simulink library "SOMANET"  (R2016b)
settings: Solver=VariableStepAuto  StartTime=0.0  StopTime=10.0  RelTol=1e-3
undefined symbols (not defined in the file): currentNominal, SomanetError
libraries: simulink x3, ConfigHandler x1, ElectricPowerMotorCalculator x1, SafetyCheckerSOMANET x1, TuningHandler x1, StatemachineSOMANET x1
settings Model: Creator=Nathan  LastModifiedBy=march

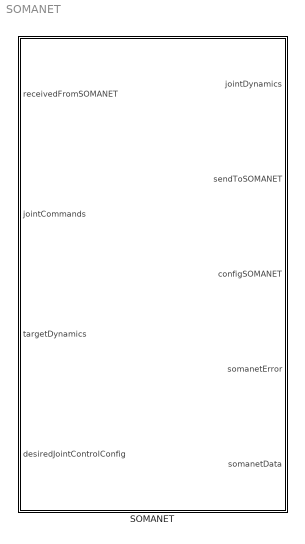
== system SOMANET ==
  SOMANET : Subsystem

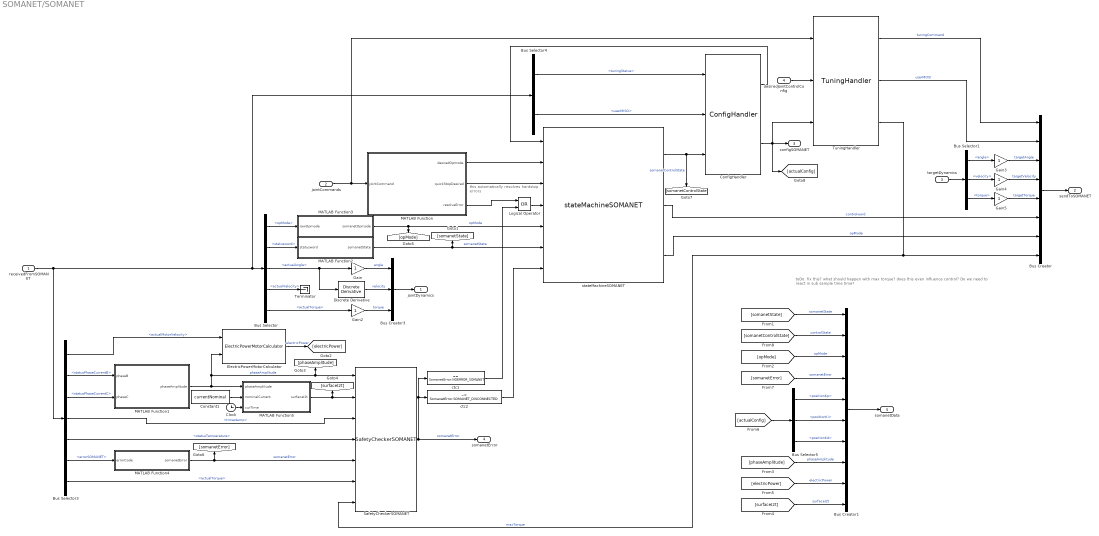
== system SOMANET/SOMANET ==
  note: this automatically resolves hardstop errors
  note: toDo: fix this? what should happen with max torque? does this even influence control? Do we need to react in sub sample time time?
  receivedFromSOMANET : Inport  OutDataTypeStr=Bus: EtherCATReceivedFromSOMANET  BusOutputAsStruct=on
  jointCommands : Inport  Port=2
  targetDynamics : Inport  Port=3  OutDataTypeStr=Bus: JointDynamics  BusOutputAsStruct=on
  desiredJointControlConfig : Inport  Port=4  OutDataTypeStr=Bus: JointControlConfig
  Bus Creator : BusCreator  Inputs=8  OutDataTypeStr=Bus: EtherCATSendToSOMANET  NonVirtualBus=on
  Bus Creator1 : BusCreator  Inputs=10  OutDataTypeStr=Bus: SOMANETData  NonVirtualBus=on
  Bus Creator3 : BusCreator  Inputs=3  OutDataTypeStr=Bus: JointDynamics  NonVirtualBus=on
  Bus Selector : BusSelector  OutputSignals=opMode,statusword,actualAngle,actualVelocity,actualTorque
  Bus Selector1 : BusSelector  OutputSignals=angle,velocity,torque
  Bus Selector3 : BusSelector  OutputSignals=actualMotorVelocity,statusPhaseCurrentB,statusPhaseCurrentC,timestamp,statusTemperature,errorSOMANET,actualTorque
  Bus Selector4 : BusSelector  OutputSignals=tuningStatus,userMISO
  Bus Selector5 : BusSelector  OutputSignals=positionKp,positionKi,positionKd
  Clock : Clock
  ConfigHandler : ConfigHandler/ConfigHandler
  Constant1 : Constant  Value=currentNominal
  Discrete Derivative : simulink/Discrete/Discrete Derivative  gainval=1.0  ICPrevScaledInput=0.0  OutMin=[]  OutMax=[]  OutDataType=fixdt(1, 16)  OutScaling=2^-10  DoSatur=off
  ElectricPowerMotorCalculator : ElectricPowerMotorCalculator/ElectricPowerMotorCalculator
  Gain{,2..5} (5 alike) : Gain
  Logical Operator : Logic  Operator=OR  AllPortsSameDT=off  OutDataTypeStr=boolean
  MATLAB Function : MATLAB Function  TreatAsAtomicUnit=on
  MATLAB Function1 : MATLAB Function  TreatAsAtomicUnit=on
  MATLAB Function2 : MATLAB Function  TreatAsAtomicUnit=on
  MATLAB Function3 : MATLAB Function  TreatAsAtomicUnit=on
  MATLAB Function4 : MATLAB Function  TreatAsAtomicUnit=on
  MATLAB Function5 : MATLAB Function  TreatAsAtomicUnit=on
  SafetyCheckerSOMANET : SafetyCheckerSOMANET/SafetyCheckerSOMANET
  Terminator : Terminator
  TuningHandler : TuningHandler/TuningHandler
  ctc1 : simulink/Logic and Bit Operations/Compare To Constant  relop===  const=SomanetError.NOERROR_SOMANET  OutDataTypeStr=boolean
  ctc2 : simulink/Logic and Bit Operations/Compare To Constant  relop=~=  const=SomanetError.SOMANET_DISCONNECTED  OutDataTypeStr=boolean
  stateMachineSOMANET : StatemachineSOMANET/stateMachineSOMANET
  jointDynamics : Outport  OutDataTypeStr=Bus: JointDynamics
  sendToSOMANET : Outport  Port=2  OutDataTypeStr=Bus: EtherCATSendToSOMANET  BusOutputAsStruct=on
  configSOMANET : Outport  Port=3  OutDataTypeStr=Bus: JointControlConfig  BusOutputAsStruct=on
  somanetError : Outport  Port=4  OutDataTypeStr=Enum: SomanetError
  somanetData : Outport  Port=5  OutDataTypeStr=Bus: SOMANETData
  wires:
  Bus Selector5/3 -> Bus Creator1/7  "<positionKd>"
  Bus Selector5/2 -> Bus Creator1/6  "<positionKi>"
  Bus Selector5/1 -> Bus Creator1/5  "<positionKp>"
  [actualConfig] -> Bus Selector5/1
  Gain5/1 -> Bus Creator/5  "targetTorque"
  Gain3/1 -> Bus Creator/3  "targetAngle"
  Gain4/1 -> Bus Creator/4  "targetVelocity"
  Bus Selector1/3 -> Gain5/1  "<torque>"
  Bus Selector1/1 -> Gain3/1  "<angle>"
  Bus Selector1/2 -> Gain4/1  "<velocity>"
  Gain2/1 -> Bus Creator3/3  "torque"
  Discrete Derivative/1 -> Bus Creator3/2  "velocity"
  Gain/1 -> Bus Creator3/1  "angle"
  Bus Selector/2 -> MATLAB Function2/1(statusword)  "<statusword>"
  Bus Selector/1 -> MATLAB Function3/1(rawOpmode)  "<opMode>"
  ConfigHandler/1 -> stateMachineSOMANET/1
  SafetyCheckerSOMANET/1 -> ctc1/1, ctc2/1, somanetError/1  "somanetError"
  jointCommands/1 -> MATLAB Function/1(jointCommand), TuningHandler/1
  Bus Creator/1 -> sendToSOMANET/1
  receivedFromSOMANET/1 -> Bus Selector4/1, Bus Selector/1, Bus Selector3/1
  TuningHandler/3 -> SafetyCheckerSOMANET/7, Bus Creator/8  "maxTorque"
  MATLAB Function3/1(somanetOpmode) -> [opMode], stateMachineSOMANET/5  "opMode"
  MATLAB Function2/1(somanetState) -> [somanetState], stateMachineSOMANET/6  "somanetState"
  MATLAB Function/1(desiredOpmode) -> stateMachineSOMANET/2
  ctc2/1 -> stateMachineSOMANET/7
  MATLAB Function/2(quickStopDesired) -> stateMachineSOMANET/3
  Bus Creator3/1 -> jointDynamics/1
  Bus Selector/4 -> Terminator/1  "<actualVelocity>"
  Bus Selector/3 -> Gain/1, Discrete Derivative/1  "<actualAngle>"
  targetDynamics/1 -> Bus Selector1/1
  Bus Selector4/1 -> ConfigHandler/1  "<tuningStatus>"
  Bus Selector4/2 -> ConfigHandler/2  "<userMISO>"
  stateMachineSOMANET/1 -> [somanetControlState], ConfigHandler/3  "somanetControlState"
  ConfigHandler/2 -> [actualConfig], configSOMANET/1, TuningHandler/3
  desiredJointControlConfig/1 -> TuningHandler/2
  TuningHandler/1 -> Bus Creator/1  "tuningCommand"
  TuningHandler/2 -> Bus Creator/2  "userMOSI"
  stateMachineSOMANET/2 -> Bus Creator/6  "controlword"
  stateMachineSOMANET/3 -> Bus Creator/7  "opMode"
  Bus Selector/5 -> Gain2/1  "<actualTorque>"
  Bus Selector3/1 -> ElectricPowerMotorCalculator/1  "<actualMotorVelocity>"
  Bus Selector3/2 -> MATLAB Function1/1(phaseB)  "<statusPhaseCurrentB>"
  Bus Selector3/3 -> MATLAB Function1/2(phaseC)  "<statusPhaseCurrentC>"
  Bus Selector3/6 -> MATLAB Function4/1(errorCode)  "<errorSOMANET>"
  MATLAB Function4/1(somanetError) -> SafetyCheckerSOMANET/5, [somanetError]  "somanetError"
  MATLAB Function1/1(phaseAmplitude) -> ElectricPowerMotorCalculator/2, [phaseAmplitude], SafetyCheckerSOMANET/1, MATLAB Function5/1(phaseAmplitude)  "phaseAmplitude"
  Clock/1 -> MATLAB Function5/3(curTime)
  MATLAB Function5/1(surfaceI2t) -> SafetyCheckerSOMANET/2, [surfaceI2t]
  Bus Selector3/4 -> SafetyCheckerSOMANET/3  "<timestamp>"
  Bus Selector3/5 -> SafetyCheckerSOMANET/4  "<statusTemperature>"
  Constant1/1 -> MATLAB Function5/2(nominalCurrent)
  ElectricPowerMotorCalculator/1 -> [electricPower]  "electricPower"
  [somanetState] -> Bus Creator1/1  "somanetState"
  [opMode] -> Bus Creator1/3  "opMode"
  [somanetError] -> Bus Creator1/4  "somanetError"
  [somanetControlState] -> Bus Creator1/2  "controlState"
  [phaseAmplitude] -> Bus Creator1/8  "phaseAmplitude"
  [electricPower] -> Bus Creator1/9  "electricPower"
  [surfaceI2t] -> Bus Creator1/10  "surfaceI2t"
  Bus Creator1/1 -> somanetData/1
  Bus Selector3/7 -> SafetyCheckerSOMANET/6  "<actualTorque>"
  Logical Operator/1 -> stateMachineSOMANET/4
  MATLAB Function/3(resolveError) -> Logical Operator/1
  ctc1/1 -> Logical Operator/2

== matlab function SOMANET/MATLAB Function5 ==
  data: phaseAmplitude input; surfaceI2t output; nominalCurrent input; curTime input
function surfaceI2t = getI2tSurface( phaseAmplitude, nominalCurrent, curTime )
% wrapper for getI2tSurface
surfaceI2t = getI2tSurface(phaseAmplitude, nominalCurrent, curTime);
end

== matlab function SOMANET/MATLAB Function ==
  data: jointCommand input; desiredOpmode output; quickStopDesired output; resolveError output
function [desiredOpmode, quickStopDesired, resolveError] = getSomanetCommands(jointCommand)
% jointCommand should be some enum
% with possible values something like:
%   * torqueControl
%   * positionControl
%   * velocityControl
%   * deactivateMotors
%   * resetError (?)
%   * don't move
% from these commands, the desired control words/opmodes/quick stops/
% whatever can be derived.
% point of this is that the master can be agnostic about the precise
% control mechanism of the somanet
persistent prevOpmode;
if(isempty(prevOpmode))
    prevOpmode = SomanetOpmode.CSTORQUE;
end

switch jointCommand
    case JointCommand.POSITIONCONTROL
        desiredOpmode = SomanetOpmode.CSPOSITION;
        quickStopDesired = 0;
        resolveError = 0;
    case JointCommand.VELOCITYCONTROL
        desiredOpmode = SomanetOpmode.CSVELOCITY;
        quickStopDesired = 0;
        resolveError = 0;
    case JointCommand.TORQUECONTROL
        desiredOpmode = SomanetOpmode.CSTORQUE;
        quickStopDesired = 0;
        resolveError = 0;
    case JointCommand.RESOLVEERROR
        desiredOpmode = prevOpmode;
        quickStopDesired = 0;
        resolveError = 1;
    case JointCommand.SYNCCONFIGS
        desiredOpmode = SomanetOpmode.TUNING;
        quickStopDesired = 0;
        resolveError = 0;
    case JointCommand.TUNECOMMUTATIONOFFSET
        desiredOpmode = SomanetOpmode.TUNING;
        quickStopDesired = 0;
        resolveError = 0;
    otherwise
        desiredOpmode = SomanetOpmode.CSTORQUE;
        quickStopDesired = 1;
        resolveError = 0;
end

% update persistent variables
prevOpmode = desiredOpmode;
end

== matlab function SOMANET/MATLAB Function1 ==
  data: phaseB input; phaseAmplitude output; phaseC input
function phaseAmplitude = getPhaseAmplitude( phaseB, phaseC )
% wrapper function for getPhaseAmplitude
[ phaseAmplitude ] = getPhaseAmplitude( phaseB, phaseC );
end

== matlab function SOMANET/MATLAB Function2 ==
  data: statusword input; somanetState output
function somanetState = getSomanetState( statusword )
% wrapper function for getSomanetState
somanetState = getSomanetState( statusword );
end

== matlab function SOMANET/MATLAB Function3 ==
  data: rawOpmode input; somanetOpmode output
function somanetOpmode   = getSomanetOpmode( rawOpmode )
% wrapper function for getSomanetOpmode
somanetOpmode = getSomanetOpmode(rawOpmode);
end

== matlab function SOMANET/MATLAB Function4 ==
  data: errorCode input; somanetError output
function somanetError  = getErrorFromErrorCode(errorCode)
% wrapper for getErrorFromErroCode
somanetError = getErrorFromErrorCode(errorCode);
end
